simulink model "System_Model_Updated_0"  (R2021a)
settings: Solver=VariableStepAuto  StartTime=0.0  StopTime=10.0  RelTol=1e-3
libraries: vrlib x1, pid_lib x1
settings Model: Creator=Hameed  LastModifiedBy=Hameed

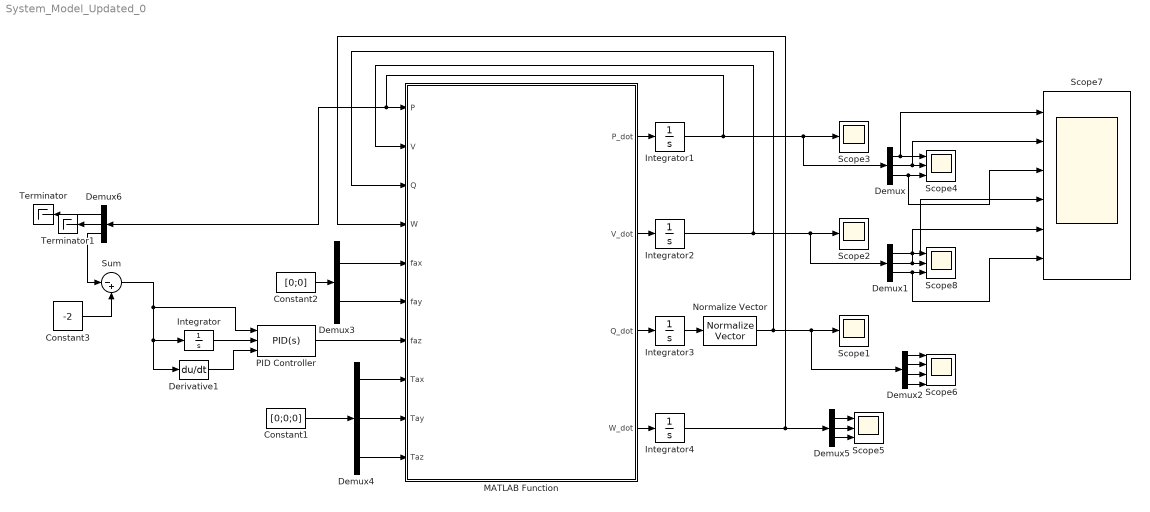
== system System_Model_Updated_0 ==
  Constant1 : Constant  Value=[0;0;0]  VectorParams1D=off
  Constant2 : Constant  Value=[0;0]  VectorParams1D=off
  Constant3 : Constant  Value=-2  VectorParams1D=off
  Demux{,1,4..6} (5 alike) : Demux  Outputs=3
  Demux2 : Demux
  Demux3 : Demux  Outputs=2
  Derivative1 : Derivative
  Integrator : Integrator
  Integrator1 : Integrator  InitialCondition=[0;0;0]
  Integrator2 : Integrator  InitialCondition=[0;0;0]
  Integrator3 : Integrator  InitialCondition=[1;0;0;0]
  Integrator4 : Integrator  InitialCondition=[0;0;0]
  MATLAB Function : MATLAB Function  TreatAsAtomicUnit=on
  Normalize Vector : vrlib/Utilities/Normalize Vector  maxzero=0
  PID Controller : pid_lib/PID Controller  Controller=PID  Form=Parallel  TimeDomain=Continuous-time  UseExternalTs=off  SampleTime=-1  IntegratorMethod=Forward Euler  FilterMethod=Forward Euler  ControllerParametersSource=internal  P=50  I=60  D=30  UseFilter=on  N=100  TunerSelectOption=Transfer Function Based (PID Tuner App)  InitialConditionSource=external  InitialConditionForIntegrator=0  InitialConditionForFilter=0  DifferentiatorICPrevScaledInput=0  ExternalReset=none  TrackingMode=off  Kt=1  LimitOutput=off  SatLimitsSource=internal  UpperSaturationLimit=inf  LowerSaturationLimit=-inf  LinearizeAsGain=on  AntiWindupMode=none  Kb=1  POutMin=[]  POutMax=[]  IOutMin=[]  IOutMax=[]  DOutMin=[]  DOutMax=[]  NOutMin=[]  NOutMax=[]  SumOutMin=[]  SumOutMax=[]  SaturationOutMin=[]  SaturationOutMax=[]  PParamMin=[]  PParamMax=[]  IParamMin=[]  IParamMax=[]  DParamMin=[]  DParamMax=[]  NParamMin=[]  NParamMax=[]  KbParamMin=[]  KbParamMax=[]  KtParamMin=[]  KtParamMax=[]  KbOutMin=[]  KbOutMax=[]  KtOutMin=[]  KtOutMax=[]  IntegratorOutMin=[]  IntegratorOutMax=[]  FilterOutMin=[]  FilterOutMax=[]  SumI1OutMin=[]  SumI1OutMax=[]  SumI2OutMin=[]  SumI2OutMax=[]  SumI3OutMin=[]  SumI3OutMax=[]  SumI4OutMin=[]  SumI4OutMax=[]  SumDOutMin=[]  SumDOutMax=[]  DifferentiatorOutMin=[]  DifferentiatorOutMax=[]  FilterDiffOutCoefMin=[]  FilterDiffOutCoefMax=[]  ReciprocalOutMin=[]  ReciprocalOutMax=[]  SumDenOutMin=[]  SumDenOutMax=[]  SumNumOutMin=[]  SumNumOutMax=[]  DivideOutMin=[]  DivideOutMax=[]  UdiffTsProdOutMin=[]  UdiffTsProdOutMax=[]  NTsProdOutMin=[]  NTsProdOutMax=[]  UintegralTsProdOutMin=[]  UintegralTsProdOutMax=[]  UngainTsProdOutMin=[]  UngainTsProdOutMax=[]  IntegratorContinuousStateAttributes=''  IntegratorStateMustResolveToSignalObject=off  IntegratorRTWStateStorageClass=Auto  FilterContinuousStateAttributes=''  FilterStateMustResolveToSignalObject=off  FilterRTWStateStorageClass=Auto  ParallelPVariant=InternalParameters  IdealPVariant=Disabled  IVariant=InternalParameters  DVariant=InternalParameters  IntegratorVariant=Continuous  SatVariant=Disabled  AWVariant=Passthrough  PCopyVariant=Disabled  TRVariant=Disabled  FdbkBlocksVariant=Forward  IdealPFdbkVariant=Disabled  SatFdbkVariant=Disabled  DerivativeFilterVariant=ContFilter  NVariant=InternalParameters  NCopyVariant=Disabled  FilterICVariant=ExternalICs  IntegratorICVariant=ExternalICs  ExternalResetVariant=Disabled  TRSumVariant=Passthrough  SumFdbkVariant=Disabled  SumVariant=Sum_PID  TsampFilterVariant=InternalTs  TsampNgainVariant=Passthrough  TsampIntegralVariant=Passthrough  ExternalSaturationOutDataTypeStr=Inherit: Same as second input
  Scope1 : Scope
  Scope2 : Scope
  Scope3 : Scope
  Scope4 : Scope  NumInputPorts=3
  Scope5 : Scope  NumInputPorts=3
  Scope6 : Scope  NumInputPorts=4
  Scope7 : Scope  NumInputPorts=6
  Scope8 : Scope  NumInputPorts=3
  Sum : Sum  Inputs=|-+
  Terminator : Terminator
  Terminator1 : Terminator
  wires:
  Integrator3/1 -> Normalize Vector/1
  Integrator1/1 -> Scope3/1, Demux/1, Demux6/1, MATLAB Function/1(P)
  Derivative1/1 -> PID Controller/3
  Demux6/3 -> Sum/1
  Integrator/1 -> PID Controller/2
  Demux2/2 -> Scope6/2
  Demux5/3 -> Scope5/3
  Constant3/1 -> Sum/2
  Demux3/1 -> MATLAB Function/5(fax)
  Sum/1 -> PID Controller/1, Derivative1/1, Integrator/1
  Demux6/2 -> Terminator1/1
  Demux2/3 -> Scope6/3
  Demux6/1 -> Terminator/1
  Demux5/1 -> Scope5/1
  Demux5/2 -> Scope5/2
  Constant2/1 -> Demux3/1
  MATLAB Function/4(W_dot) -> Integrator4/1
  MATLAB Function/1(P_dot) -> Integrator1/1
  Demux1/2 -> Scope7/5, Scope8/2
  Demux2/4 -> Scope6/4
  Integrator2/1 -> Demux1/1, Scope2/1, MATLAB Function/2(V)
  Demux/3 -> Scope7/3, Scope4/3
  Integrator4/1 -> Demux5/1, MATLAB Function/4(W)
  MATLAB Function/2(V_dot) -> Integrator2/1
  Demux1/1 -> Scope7/4, Scope8/1
  Demux/2 -> Scope7/2, Scope4/2
  Demux/1 -> Scope4/1, Scope7/1
  Demux2/1 -> Scope6/1
  PID Controller/1 -> MATLAB Function/7(faz)
  Demux3/2 -> MATLAB Function/6(fay)
  MATLAB Function/3(Q_dot) -> Integrator3/1
  Demux1/3 -> Scope7/6, Scope8/3
  Demux4/2 -> MATLAB Function/9(Tay)
  Demux4/1 -> MATLAB Function/8(Tax)
  Demux4/3 -> MATLAB Function/10(Taz)
  Constant1/1 -> Demux4/1
  Normalize Vector/1 -> Scope1/1, Demux2/1, MATLAB Function/3(Q)

== matlab function System_Model_Updated_0/MATLAB Function ==
  data: P input; P_dot output; V input; Q input; W input; V_dot output; Q_dot output; W_dot output; fax input; fay input; faz input; Tax input; Tay input; Taz input
function [P_dot,V_dot,Q_dot,W_dot]= fcn(P,V,Q,W,fax,fay,faz,Tax,Tay,Taz)
clc
m=5;

%%% phi=Q(2); % theta=Q(3); % psi=Q(4);

% Rz=[cos(psi) sin(psi) 0;-sin(psi)) cos(psi) 0;0 0 1];
% Rx=[1 0 0;0 cos(phi) sin(phi);0 -sin(phi) cos(phi)];
% Ry=[cos(theta) 0 -sin(theta);0 1 0;sin(theta) 0 cos(theta)];

Rz=[cos(Q(4)) sin(Q(4)) 0; -sin(Q(4)) cos(Q(4)) 0; 0 0 1];
Rx=[1 0 0; 0 cos(Q(2)) sin(Q(2)); 0 -sin(Q(2)) cos(Q(2))];
Ry=[cos(Q(3)) 0 -sin(Q(3)); 0 1 0; sin(Q(3)) 0 cos(Q(3))];

Rb=Rz*Ry*Rx;
Rs=[1 0 0;
    0 0 -1;
    0 1 0 ];

%Rs=[1 0 0;0 -1 0;0 0 -1];
%lambda=L;
L=0;
%L=1;
Rd=[1 0 0;
    0 1 0;
    0 0 1-L];

SL=Rs*Rd*transpose(Rs);

rT=[0.5;0;0];

Ixx=1;
Iyy=1;
Izz=1;
J=[Ixx 0 0;0 Iyy 0;0 0 Izz];

g=9.8;
dF=[0;0;0];
fc=[0;0;0];
rcom=[0;0;0];
dT=[0;0;0];

fa=[fax;fay;faz];
ta=[Tax;Tay;Taz];

ab=(m^-1)*((Rb*fa)+(L*fc)+dF)+[0;0;g];

% T=[0 -sin(Q(2)) cos(Q(2))*sin(Q(3));
% 0 cos(Q(2)) sin(Q(2))*sin(Q(3));
% 1 0 cos(Q(3))];

Sq=[0 -Q(4) Q(3);
    Q(4) 0 -Q(2);
    -Q(3) Q(2) 0];

eata_dot=[Q(2);Q(3);Q(4)]
%w=T*eata_dot;

h=J*W;
h1=transpose(Rb)*[0;0;m*g];
h2=L*transpose(Rb)*fc;

P_dot=SL*V;

Qw_dot=-1/2*[Q(2) Q(3) Q(4)]*W;
Qv_dot=1/2*(Q(1)*J-Sq)*W;

% Qw_dot=-1/2*[Q(2) Q(3) Q(4)]*W
% Qv_dot=1/2*(Q(1)*J-Sq)*W;
Q_dot=[Qw_dot;Qv_dot];

W_dot=(inv(J))*(ta-cross(W,h)+cross(rcom,h1)+cross(rT,h2)+dT);

V_dot=SL*((ab)+Rb*(cross(W_dot,rT)+(cross(W,cross(W,rT)))));
